simulink model "untitled"  (R2019b)
settings: Solver=VariableStepAuto  StartTime=0.0  StopTime=30  RelTol=1e-3
settings Model: Creator=Lenovo  LastModifiedBy=Lenovo

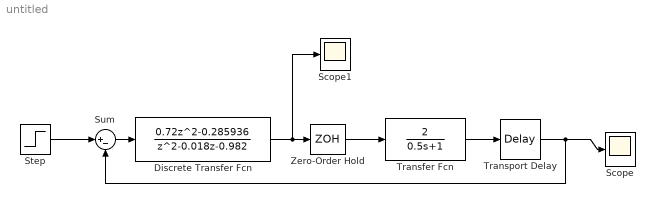
== system untitled ==
  Discrete Transfer Fcn : DiscreteTransferFcn  Numerator=[0.72 0 -0.285936]  Denominator=[1 -0.018 -0.982]
  Scope : Scope
  Scope1 : Scope
  Step : Step  SampleTime=0
  Sum : Sum  Inputs=|+-
  Transfer Fcn : TransferFcn  Numerator=[2]  Denominator=[0.5 1]
  Transport Delay : TransportDelay  DelayTime=0.5
  Zero-Order Hold : ZeroOrderHold  SampleTime=0.5
  wires:
  Discrete Transfer Fcn/1 -> Scope1/1, Zero-Order Hold/1
  Zero-Order Hold/1 -> Transfer Fcn/1
  Transfer Fcn/1 -> Transport Delay/1
  Transport Delay/1 -> Sum/2, Scope/1
  Sum/1 -> Discrete Transfer Fcn/1
  Step/1 -> Sum/1
